simulink model "variableintegerdelay_tut"  (Simulink 5.0)
settings: Solver=FixedStepDiscrete  StartTime=0.0  StopTime=5  RelTol=1e-3
libraries: dspsrcs4 x2, dspsigops x1
settings Model: Creator=ckamachi  LastModifiedBy=ckamachi  ExtModeTrigMode=oneshot  ExtModeArmWhenConnect=off  LimitDataPoints=off  BlockReductionOpt=off  BooleanDataType=off

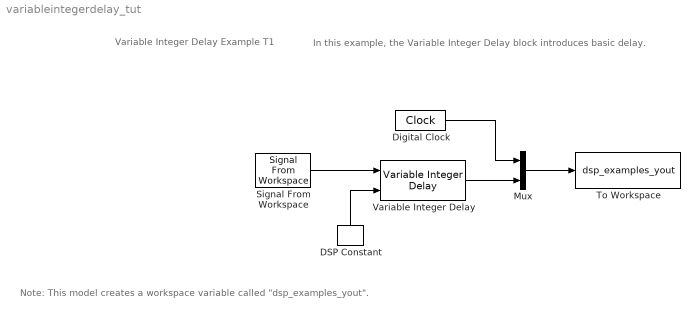
== system variableintegerdelay_tut ==
  note: Variable Integer Delay Example T1
  note: In this example, the Variable Integer Delay block
      | introduces basic delay.
  note: Note: This model creates a workspace variable called "dsp_examples_yout".
  DSP Constant : dspsrcs4/DSP Constant  Orientation=up  Value=3  SampleMode=Discrete  discreteOutput=Sample-based  continuousOutput=Sample-based  sampTime=1  framePeriod=1  dataType=Inherit from 'Constant value'  wordLen=16  udDataType=sfix(16)  fracBitsMode=Best precision  numFracBits=15  InterpretAs1D=off  Ts=1  FramebasedOutput=off
  Digital Clock : DigitalClock
  Mux : Mux  Inputs=2
  Signal From Workspace : dspsrcs4/Signal From Workspace  X=1:100  Ts=1  nsamps=1  OutputAfterFinalValue=Setting to zero
  To Workspace : ToWorkspace  VariableName=dsp_examples_yout  SampleTime=-1  SaveFormat=Array
  Variable Integer Delay : dspsigops/Variable Integer Delay  dmax=100  ic=-1
  wires:
  Mux/1 -> To Workspace/1
  Variable Integer Delay/1 -> Mux/2
  Signal From Workspace/1 -> Variable Integer Delay/1
  Digital Clock/1 -> Mux/1
  DSP Constant/1 -> Variable Integer Delay/2
